simulink model "velocity_model"  (R2019b)
settings: Solver=VariableStepAuto  StartTime=0.0  StopTime=30.0  RelTol=1e-9
undefined symbols (not defined in the file): x_0
settings Model: Creator=Charlie  LastModifiedBy=Charlie

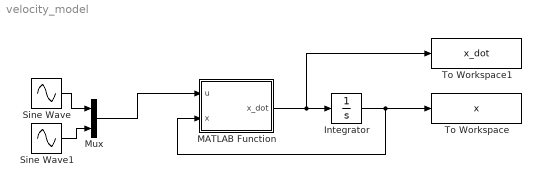
== system velocity_model ==
  Integrator : Integrator  InitialCondition=x_0
  MATLAB Function : MATLAB Function  TreatAsAtomicUnit=on
  Mux : Mux  Inputs=2
  Sine Wave : Sin  Amplitude=.2  SampleTime=0
  Sine Wave1 : Sin  Amplitude=.2  Phase=pi/2  SampleTime=0
  To Workspace : ToWorkspace  VariableName=x  SampleTime=-1
  To Workspace1 : ToWorkspace  VariableName=x_dot  SampleTime=-1
  wires:
  MATLAB Function/1(x_dot) -> To Workspace1/1, Integrator/1
  Integrator/1 -> To Workspace/1, MATLAB Function/2(x)
  Sine Wave/1 -> Mux/1
  Sine Wave1/1 -> Mux/2
  Mux/1 -> MATLAB Function/1(u)

== matlab function velocity_model/MATLAB Function ==
  data: u input; x_dot output; x input; P parameter
function x_dot = EOM(u, x, P)
theta   = x(1:2);
phi     = x(3:4);

M = zeros(10);
b = zeros(10,1);
% Row 1
M(1,4) = P.a4*sin(phi(2)) - P.c4*cos(phi(2));
M(1,5) = 1;
% Row 2
M(2,1) =-P.r2*sin(theta(1));
M(2,3) =-P.a4*cos(phi(1))*sin(phi(2)) + P.c4*cos(phi(1))*cos(phi(2));
M(2,4) =-P.a4*sin(phi(1))*cos(phi(2)) - P.c4*cos(phi(1))*sin(phi(2));
M(2,6) = 1;
% Row 3
M(3,1) = P.r2*cos(theta(1));
M(3,3) =-P.a4*sin(phi(1))*sin(phi(2)) + P.c4*sin(phi(1))*cos(phi(2));
M(3,4) = P.a4*cos(phi(1))*cos(phi(2)) + P.c4*cos(phi(1))*sin(phi(2));
M(3,7) = 1;
% Row 4
M(4,5) = x(5);
M(4,6) = x(6);
M(4,7) = x(7);
% Row 5
M(5,2) = P.r6*sin(theta(2));
M(5,4) =-P.c8*cos(phi(2));
M(5,8) = 1;
% Row 6
M(6,3) = P.b8*sin(phi(1)) + P.c8*cos(phi(1))*cos(phi(2));
M(6,4) =-P.c8*sin(phi(1))*sin(phi(2));
M(6,9) = 1;
% Row 7
M(7,2) = P.r6*cos(theta(2));
M(7,3)  =-P.b8*cos(phi(1)) + P.c8*sin(phi(1))*cos(phi(2));
M(7,4)  = P.c8*cos(phi(1))*sin(phi(2));
M(7,10) = 1;
% Row 8
M(8,8)  = x(8);
M(8,9)  = x(9);
M(8,10) = x(10);
% Row 9
M(9,1) = 1;
b(9) = u(1);
% Row 10
M(10,2) = 1;
b(10) = u(2);
%
x_dot = M\b;
end
